simulink model "Electron_Energization_Index2"  (R2015a)
settings: Solver=ode45  StartTime=0.0  StopTime=5000  RelTol=1e-3
values from neighbouring files (symbols this model uses):
  t_delay_E_index = 10    [test_2taus.m]    (also in windmi.m = 0)
settings Model: CovSFcnEnable=off  Creator=edmund  LastModifiedBy=Pavithra
settings DataIOCC: LimitDataPoints=off  InspectSignalLogs=on  TimeSaveName=tout_E  OutputSaveName=yout_E

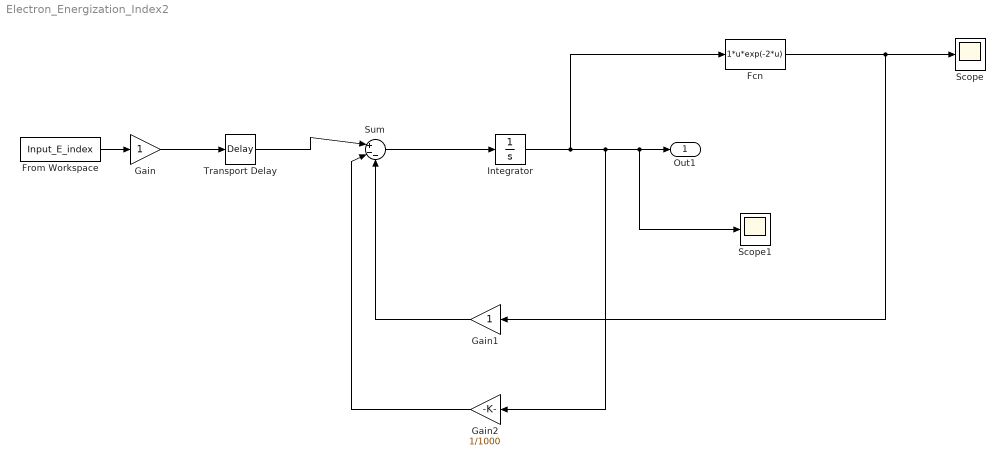
== system Electron_Energization_Index2 ==
  Fcn : Fcn  Expr=1*u*exp(-2*u)
  From Workspace : FromWorkspace  VariableName=Input_E_index  SampleTime=0
  Gain : Gain
  Gain1 : Gain
  Gain2 : Gain  Gain=1/1000
  Integrator : Integrator
  Scope : Scope
  Scope1 : Scope
  Sum : Sum  Inputs=|+--
  Transport Delay : TransportDelay  DelayTime=t_delay_E_index
  Out1 : Outport
  wires:
  From Workspace/1 -> Gain/1
  Gain/1 -> Transport Delay/1
  Transport Delay/1 -> Sum/1
  Gain1/1 -> Sum/3
  Sum/1 -> Integrator/1
  Integrator/1 -> Fcn/1, Gain2/1, Scope1/1, Out1/1
  Fcn/1 -> Gain1/1, Scope/1
  Gain2/1 -> Sum/2
